simulink model "BigFour6sStEnCtrl"  (R2018b)
settings: Solver=FixedStepDiscrete  StartTime=0.0  StopTime=10.0  RelTol=1e-3
undefined symbols (not defined in the file or in its folder): data, KeSMSw4SSecRwLtStLgrstOtwdInwdClosePos1_Val, KeSMSw4SSecRwLtStLgrstUpwdDnwdClosePos1_Val, KeSMSw4SSecRwLtStLgrstUpwdDnwdClosePos2_Val, SecRwLtStBkReclnEn_Clear, SecRwLtStBkReclnEn_Set, SecRwLtStFwdBkwdEn_Clear, SecRwLtStFwdBkwdEn_Set, SecRwLtStLgrstInwdOtwdEn_Clear, SecRwLtStLgrstInwdOtwdEn_Set, SecRwLtStLgrstUpwdDnwdEn_Clear, SecRwLtStLgrstUpwdDnwdEn_Set, SecRwRtStBkReclnEn_Clear, SecRwRtStBkReclnEn_Set, SecRwRtStFwdBkwdEn_Clear, SecRwRtStFwdBkwdEn_Set, SecRwRtStLgrstInwdOtwdEn_Clear, SecRwRtStLgrstInwdOtwdEn_Set, SecRwRtStLgrstUpwdDnwdEn_Clear, SecRwRtStLgrstUpwdDnwdEn_Set, ThdRwLtStBkReclnEn_Clear, ThdRwLtStBkReclnEn_Set, ThdRwLtStFwdBkwdEn_Clear, ThdRwLtStFwdBkwdEn_Set, ThdRwRtStBkReclnEn_Clear, ThdRwRtStBkReclnEn_Set, ThdRwRtStFwdBkwdEn_Clear, ThdRwRtStFwdBkwdEn_Set, ZeroLEn_Clear, ZeroLEn_Set, ZeroREn_Clear, ZeroREn_Set
libraries: simulink x1
settings Model: Creator=sn2xws  LastModifiedBy=sn55gm
settings Model: ModifiedHistory=|
  | 2024.9.9 V3.0.0 新增Md56
  | 2024.9.26 V3.0.1 Md56流程从Md1复制
settings DataIOCC: SaveFormat=StructureWithTime
settings OptimizationCC: DefaultParameterBehavior=Inlined  EnhancedBackFolding=on  PassReuseOutputArgsAs=Individual arguments  ZeroExternalMemoryAtStartup=off  ZeroInternalMemoryAtStartup=off  OptimizeBlockOrder=speed  DifferentSizesBufferReuse=on  OptimizationCustomize=off
settings DebuggingCC: ParameterTunabilityLossMsg=error
settings SFSimCC: MATLABDynamicMemAlloc=off
settings RTWCC: SystemTargetFile=autosar.tlc  GenCodeOnly=on  TemplateMakefile=ert_default_tmf  Description=AUTOSAR  GenerateReport=on  IncludeHyperlinkInReport=on  LaunchReport=on  GenerateTraceInfo=on  GenerateTraceReport=on  GenerateTraceReportSl=on  GenerateTraceReportSf=on  GenerateTraceReportEml=on
settings CodeAppCC: ForceParamTrailComments=on  IgnoreCustomStorageClasses=off  OperatorAnnotations=on  SimulinkDataObjDesc=on  SFDataObjDesc=on  InsertBlockDesc=on
settings STFCustomTargetCC: TargetLangStandard=C99 (ISO)  MultiwordLength=256  ParMdlRefBuildCompliant=on  CompOptLevelCompliant=on  IncludeMdlTerminateFcn=off  CombineOutputUpdateFcns=on  SuppressErrorStatus=on  ERTCustomFileBanners=on  SupportNonFinite=off  SupportComplex=off  SupportContinuousTime=off  SupportNonInlinedSFcns=off  RemoveResetFunc=on  MATLABClassNameForMDSCustomization=Simulink.SoftwareTarget.ERTCustomization  AutosarCompliant=on  UseToolchainInfoCompliant=on  LookupTableObjectStructAxisOrder=2,1,3,4,...  LUTObjectStructOrderEvenSpacing=Size,Table,Breakpoints  SystemTargetFile=autosar.tlc
settings ERTTargetCC: TargetLangStandard=C99 (ISO)  ConcurrentExecutionCompliant=off  IncludeMdlTerminateFcn=off  SuppressErrorStatus=on  SupportNonFinite=off  SupportComplex=off  ModelStepFunctionPrototypeControlCompliant=off  CPPClassGenCompliant=off  AutosarCompliant=on  LookupTableObjectStructAxisOrder=2,1,3,4,...  LUTObjectStructOrderEvenSpacing=Size,Table,Breakpoints  InlinedParameterPlacement=NonHierarchical  ERTCustomFileTemplate=example_file_process.tlc  ERTFilePackagingFormat=Compact

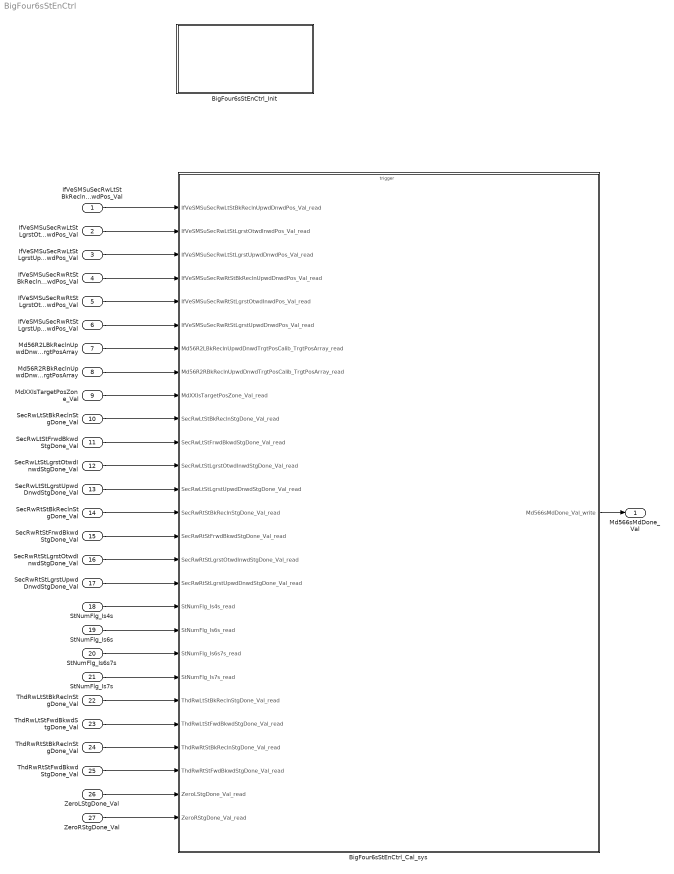
== system BigFour6sStEnCtrl ==
  IfVeSMSuSecRwLtStBkReclnUpwdDnwdPos_Val : Inport  OutDataTypeStr=uint16  PortDimensions=1
  IfVeSMSuSecRwLtStLgrstOtwdInwdPos_Val : Inport  Port=2  OutDataTypeStr=uint16  PortDimensions=1
  IfVeSMSuSecRwLtStLgrstUpwdDnwdPos_Val : Inport  Port=3  OutDataTypeStr=uint16  PortDimensions=1
  IfVeSMSuSecRwRtStBkReclnUpwdDnwdPos_Val : Inport  Port=4  OutDataTypeStr=uint16  PortDimensions=1
  IfVeSMSuSecRwRtStLgrstOtwdInwdPos_Val : Inport  Port=5  OutDataTypeStr=uint16  PortDimensions=1
  IfVeSMSuSecRwRtStLgrstUpwdDnwdPos_Val : Inport  Port=6  OutDataTypeStr=uint16  PortDimensions=1
  Md56R2LBkReclnUpwdDnwdTrgtPosCalib_TrgtPosArray : Inport  Description=|  Port=7  OutDataTypeStr=uint16  PortDimensions=3
      | 0:Pos
      | 1:Max
      | 2:Min
  Md56R2RBkReclnUpwdDnwdTrgtPosCalib_TrgtPosArray : Inport  Description=|  Port=8  OutDataTypeStr=uint16  PortDimensions=3
      | 0:Pos
      | 1:Max
      | 2:Min
  MdXXIsTargetPosZone_Val : Inport  Port=9  OutDataTypeStr=uint32  PortDimensions=1
  SecRwLtStBkReclnStgDone_Val : Inport  Port=10  OutDataTypeStr=boolean  PortDimensions=1
  SecRwLtStFrwdBkwdStgDone_Val : Inport  Port=11  OutDataTypeStr=boolean  PortDimensions=1
  SecRwLtStLgrstOtwdInwdStgDone_Val : Inport  Port=12  OutDataTypeStr=boolean  PortDimensions=1
  SecRwLtStLgrstUpwdDnwdStgDone_Val : Inport  Port=13  OutDataTypeStr=boolean  PortDimensions=1
  SecRwRtStBkReclnStgDone_Val : Inport  Port=14  OutDataTypeStr=boolean  PortDimensions=1
  SecRwRtStFrwdBkwdStgDone_Val : Inport  Port=15  OutDataTypeStr=boolean  PortDimensions=1
  SecRwRtStLgrstOtwdInwdStgDone_Val : Inport  Port=16  OutDataTypeStr=boolean  PortDimensions=1
  SecRwRtStLgrstUpwdDnwdStgDone_Val : Inport  Port=17  OutDataTypeStr=boolean  PortDimensions=1
  StNumFlg_Is4s : Inport  Port=18  OutDataTypeStr=boolean  PortDimensions=1
  StNumFlg_Is6s : Inport  Port=19  OutDataTypeStr=boolean  PortDimensions=1
  StNumFlg_Is6s7s : Inport  Port=20  OutDataTypeStr=boolean  PortDimensions=1
  StNumFlg_Is7s : Inport  Port=21  OutDataTypeStr=boolean  PortDimensions=1
  ThdRwLtStBkReclnStgDone_Val : Inport  Port=22  OutDataTypeStr=boolean  PortDimensions=1
  ThdRwLtStFwdBkwdStgDone_Val : Inport  Port=23  OutDataTypeStr=boolean  PortDimensions=1
  ThdRwRtStBkReclnStgDone_Val : Inport  Port=24  OutDataTypeStr=boolean  PortDimensions=1
  ThdRwRtStFwdBkwdStgDone_Val : Inport  Port=25  OutDataTypeStr=boolean  PortDimensions=1
  ZeroLStgDone_Val : Inport  Port=26  OutDataTypeStr=boolean  PortDimensions=1
  ZeroRStgDone_Val : Inport  Port=27  OutDataTypeStr=boolean  PortDimensions=1
  BigFour6sStEnCtrl_Cal_sys : Subsystem
  BigFour6sStEnCtrl_Init : Subsystem
  Md566sMdDone_Val : Outport  OutDataTypeStr=uint8  PortDimensions=1
  wires:
  IfVeSMSuSecRwLtStBkReclnUpwdDnwdPos_Val/1 -> BigFour6sStEnCtrl_Cal_sys/1(IfVeSMSuSecRwLtStBkReclnUpwdDnwdPos_Val_read)
  IfVeSMSuSecRwLtStLgrstOtwdInwdPos_Val/1 -> BigFour6sStEnCtrl_Cal_sys/2(IfVeSMSuSecRwLtStLgrstOtwdInwdPos_Val_read)
  IfVeSMSuSecRwLtStLgrstUpwdDnwdPos_Val/1 -> BigFour6sStEnCtrl_Cal_sys/3(IfVeSMSuSecRwLtStLgrstUpwdDnwdPos_Val_read)
  IfVeSMSuSecRwRtStBkReclnUpwdDnwdPos_Val/1 -> BigFour6sStEnCtrl_Cal_sys/4(IfVeSMSuSecRwRtStBkReclnUpwdDnwdPos_Val_read)
  IfVeSMSuSecRwRtStLgrstOtwdInwdPos_Val/1 -> BigFour6sStEnCtrl_Cal_sys/5(IfVeSMSuSecRwRtStLgrstOtwdInwdPos_Val_read)
  IfVeSMSuSecRwRtStLgrstUpwdDnwdPos_Val/1 -> BigFour6sStEnCtrl_Cal_sys/6(IfVeSMSuSecRwRtStLgrstUpwdDnwdPos_Val_read)
  Md56R2LBkReclnUpwdDnwdTrgtPosCalib_TrgtPosArray/1 -> BigFour6sStEnCtrl_Cal_sys/7(Md56R2LBkReclnUpwdDnwdTrgtPosCalib_TrgtPosArray_read)
  Md56R2RBkReclnUpwdDnwdTrgtPosCalib_TrgtPosArray/1 -> BigFour6sStEnCtrl_Cal_sys/8(Md56R2RBkReclnUpwdDnwdTrgtPosCalib_TrgtPosArray_read)
  MdXXIsTargetPosZone_Val/1 -> BigFour6sStEnCtrl_Cal_sys/9(MdXXIsTargetPosZone_Val_read)
  SecRwLtStBkReclnStgDone_Val/1 -> BigFour6sStEnCtrl_Cal_sys/10(SecRwLtStBkReclnStgDone_Val_read)
  SecRwLtStFrwdBkwdStgDone_Val/1 -> BigFour6sStEnCtrl_Cal_sys/11(SecRwLtStFrwdBkwdStgDone_Val_read)
  SecRwLtStLgrstOtwdInwdStgDone_Val/1 -> BigFour6sStEnCtrl_Cal_sys/12(SecRwLtStLgrstOtwdInwdStgDone_Val_read)
  SecRwLtStLgrstUpwdDnwdStgDone_Val/1 -> BigFour6sStEnCtrl_Cal_sys/13(SecRwLtStLgrstUpwdDnwdStgDone_Val_read)
  SecRwRtStBkReclnStgDone_Val/1 -> BigFour6sStEnCtrl_Cal_sys/14(SecRwRtStBkReclnStgDone_Val_read)
  SecRwRtStFrwdBkwdStgDone_Val/1 -> BigFour6sStEnCtrl_Cal_sys/15(SecRwRtStFrwdBkwdStgDone_Val_read)
  SecRwRtStLgrstOtwdInwdStgDone_Val/1 -> BigFour6sStEnCtrl_Cal_sys/16(SecRwRtStLgrstOtwdInwdStgDone_Val_read)
  SecRwRtStLgrstUpwdDnwdStgDone_Val/1 -> BigFour6sStEnCtrl_Cal_sys/17(SecRwRtStLgrstUpwdDnwdStgDone_Val_read)
  StNumFlg_Is4s/1 -> BigFour6sStEnCtrl_Cal_sys/18(StNumFlg_Is4s_read)
  StNumFlg_Is6s/1 -> BigFour6sStEnCtrl_Cal_sys/19(StNumFlg_Is6s_read)
  StNumFlg_Is6s7s/1 -> BigFour6sStEnCtrl_Cal_sys/20(StNumFlg_Is6s7s_read)
  StNumFlg_Is7s/1 -> BigFour6sStEnCtrl_Cal_sys/21(StNumFlg_Is7s_read)
  ThdRwLtStBkReclnStgDone_Val/1 -> BigFour6sStEnCtrl_Cal_sys/22(ThdRwLtStBkReclnStgDone_Val_read)
  ThdRwLtStFwdBkwdStgDone_Val/1 -> BigFour6sStEnCtrl_Cal_sys/23(ThdRwLtStFwdBkwdStgDone_Val_read)
  ThdRwRtStBkReclnStgDone_Val/1 -> BigFour6sStEnCtrl_Cal_sys/24(ThdRwRtStBkReclnStgDone_Val_read)
  ThdRwRtStFwdBkwdStgDone_Val/1 -> BigFour6sStEnCtrl_Cal_sys/25(ThdRwRtStFwdBkwdStgDone_Val_read)
  ZeroLStgDone_Val/1 -> BigFour6sStEnCtrl_Cal_sys/26(ZeroLStgDone_Val_read)
  ZeroRStgDone_Val/1 -> BigFour6sStEnCtrl_Cal_sys/27(ZeroRStgDone_Val_read)
  BigFour6sStEnCtrl_Cal_sys/1(Md566sMdDone_Val_write) -> Md566sMdDone_Val/1

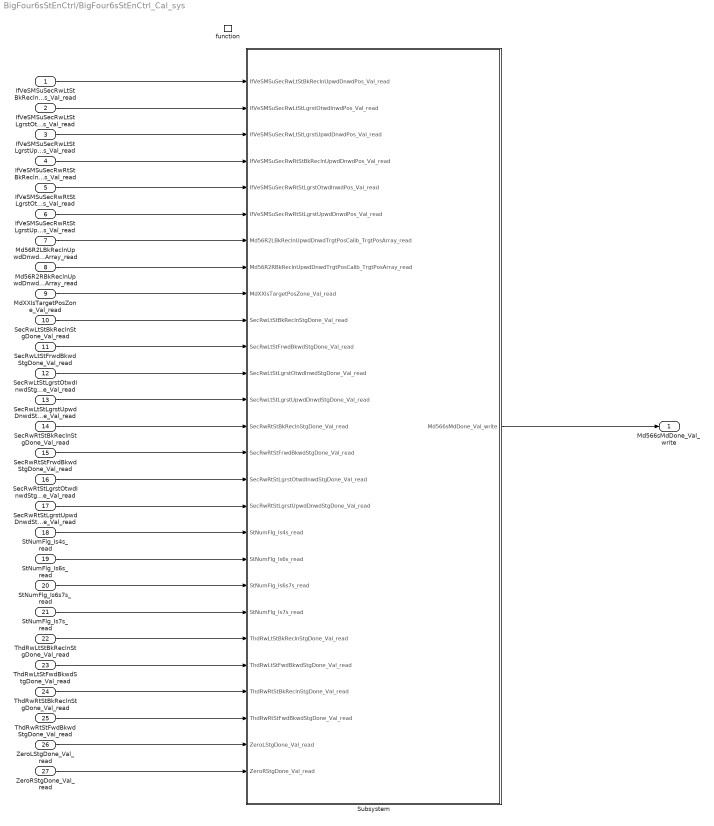
== system BigFour6sStEnCtrl/BigFour6sStEnCtrl_Cal_sys ==
  IfVeSMSuSecRwLtStBkReclnUpwdDnwdPos_Val_read : Inport
  IfVeSMSuSecRwLtStLgrstOtwdInwdPos_Val_read : Inport  Port=2
  IfVeSMSuSecRwLtStLgrstUpwdDnwdPos_Val_read : Inport  Port=3
  IfVeSMSuSecRwRtStBkReclnUpwdDnwdPos_Val_read : Inport  Port=4
  IfVeSMSuSecRwRtStLgrstOtwdInwdPos_Val_read : Inport  Port=5
  IfVeSMSuSecRwRtStLgrstUpwdDnwdPos_Val_read : Inport  Port=6
  Md56R2LBkReclnUpwdDnwdTrgtPosCalib_TrgtPosArray_read : Inport  Port=7
  Md56R2RBkReclnUpwdDnwdTrgtPosCalib_TrgtPosArray_read : Inport  Port=8
  MdXXIsTargetPosZone_Val_read : Inport  Port=9
  SecRwLtStBkReclnStgDone_Val_read : Inport  Port=10
  SecRwLtStFrwdBkwdStgDone_Val_read : Inport  Port=11
  SecRwLtStLgrstOtwdInwdStgDone_Val_read : Inport  Port=12
  SecRwLtStLgrstUpwdDnwdStgDone_Val_read : Inport  Port=13
  SecRwRtStBkReclnStgDone_Val_read : Inport  Port=14
  SecRwRtStFrwdBkwdStgDone_Val_read : Inport  Port=15
  SecRwRtStLgrstOtwdInwdStgDone_Val_read : Inport  Port=16
  SecRwRtStLgrstUpwdDnwdStgDone_Val_read : Inport  Port=17
  StNumFlg_Is4s_read : Inport  Port=18
  StNumFlg_Is6s_read : Inport  Port=19
  StNumFlg_Is6s7s_read : Inport  Port=20
  StNumFlg_Is7s_read : Inport  Port=21
  ThdRwLtStBkReclnStgDone_Val_read : Inport  Port=22
  ThdRwLtStFwdBkwdStgDone_Val_read : Inport  Port=23
  ThdRwRtStBkReclnStgDone_Val_read : Inport  Port=24
  ThdRwRtStFwdBkwdStgDone_Val_read : Inport  Port=25
  ZeroLStgDone_Val_read : Inport  Port=26
  ZeroRStgDone_Val_read : Inport  Port=27
  function : TriggerPort  TriggerType=function-call  IsSimulinkFunction=on  FunctionName=BigFour6sStEnCtrl_Cal  VariantControl=(inherit)
  Subsystem : Subsystem
  Md566sMdDone_Val_write : Outport
      settings: EnsureOutportIsVirtual=on
  wires:
  IfVeSMSuSecRwLtStBkReclnUpwdDnwdPos_Val_read/1 -> Subsystem/1(IfVeSMSuSecRwLtStBkReclnUpwdDnwdPos_Val_read)
  IfVeSMSuSecRwLtStLgrstOtwdInwdPos_Val_read/1 -> Subsystem/2(IfVeSMSuSecRwLtStLgrstOtwdInwdPos_Val_read)
  IfVeSMSuSecRwLtStLgrstUpwdDnwdPos_Val_read/1 -> Subsystem/3(IfVeSMSuSecRwLtStLgrstUpwdDnwdPos_Val_read)
  IfVeSMSuSecRwRtStBkReclnUpwdDnwdPos_Val_read/1 -> Subsystem/4(IfVeSMSuSecRwRtStBkReclnUpwdDnwdPos_Val_read)
  IfVeSMSuSecRwRtStLgrstOtwdInwdPos_Val_read/1 -> Subsystem/5(IfVeSMSuSecRwRtStLgrstOtwdInwdPos_Val_read)
  IfVeSMSuSecRwRtStLgrstUpwdDnwdPos_Val_read/1 -> Subsystem/6(IfVeSMSuSecRwRtStLgrstUpwdDnwdPos_Val_read)
  Md56R2LBkReclnUpwdDnwdTrgtPosCalib_TrgtPosArray_read/1 -> Subsystem/7(Md56R2LBkReclnUpwdDnwdTrgtPosCalib_TrgtPosArray_read)
  Md56R2RBkReclnUpwdDnwdTrgtPosCalib_TrgtPosArray_read/1 -> Subsystem/8(Md56R2RBkReclnUpwdDnwdTrgtPosCalib_TrgtPosArray_read)
  MdXXIsTargetPosZone_Val_read/1 -> Subsystem/9(MdXXIsTargetPosZone_Val_read)
  SecRwLtStBkReclnStgDone_Val_read/1 -> Subsystem/10(SecRwLtStBkReclnStgDone_Val_read)
  SecRwLtStFrwdBkwdStgDone_Val_read/1 -> Subsystem/11(SecRwLtStFrwdBkwdStgDone_Val_read)
  SecRwLtStLgrstOtwdInwdStgDone_Val_read/1 -> Subsystem/12(SecRwLtStLgrstOtwdInwdStgDone_Val_read)
  SecRwLtStLgrstUpwdDnwdStgDone_Val_read/1 -> Subsystem/13(SecRwLtStLgrstUpwdDnwdStgDone_Val_read)
  SecRwRtStBkReclnStgDone_Val_read/1 -> Subsystem/14(SecRwRtStBkReclnStgDone_Val_read)
  SecRwRtStFrwdBkwdStgDone_Val_read/1 -> Subsystem/15(SecRwRtStFrwdBkwdStgDone_Val_read)
  SecRwRtStLgrstOtwdInwdStgDone_Val_read/1 -> Subsystem/16(SecRwRtStLgrstOtwdInwdStgDone_Val_read)
  SecRwRtStLgrstUpwdDnwdStgDone_Val_read/1 -> Subsystem/17(SecRwRtStLgrstUpwdDnwdStgDone_Val_read)
  StNumFlg_Is4s_read/1 -> Subsystem/18(StNumFlg_Is4s_read)
  StNumFlg_Is6s_read/1 -> Subsystem/19(StNumFlg_Is6s_read)
  StNumFlg_Is6s7s_read/1 -> Subsystem/20(StNumFlg_Is6s7s_read)
  StNumFlg_Is7s_read/1 -> Subsystem/21(StNumFlg_Is7s_read)
  ThdRwLtStBkReclnStgDone_Val_read/1 -> Subsystem/22(ThdRwLtStBkReclnStgDone_Val_read)
  ThdRwLtStFwdBkwdStgDone_Val_read/1 -> Subsystem/23(ThdRwLtStFwdBkwdStgDone_Val_read)
  ThdRwRtStBkReclnStgDone_Val_read/1 -> Subsystem/24(ThdRwRtStBkReclnStgDone_Val_read)
  ThdRwRtStFwdBkwdStgDone_Val_read/1 -> Subsystem/25(ThdRwRtStFwdBkwdStgDone_Val_read)
  ZeroLStgDone_Val_read/1 -> Subsystem/26(ZeroLStgDone_Val_read)
  ZeroRStgDone_Val_read/1 -> Subsystem/27(ZeroRStgDone_Val_read)
  Subsystem/1(Md566sMdDone_Val_write) -> Md566sMdDone_Val_write/1

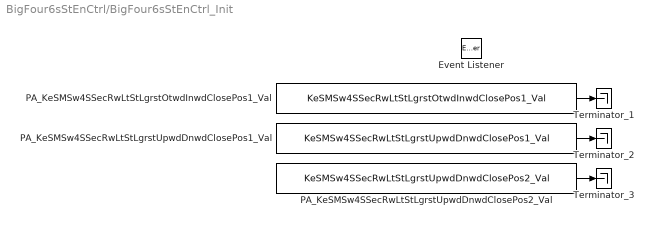
== system BigFour6sStEnCtrl/BigFour6sStEnCtrl_Init ==
  Event Listener : EventListener  EventName=reset
  PA_KeSMSw4SSecRwLtStLgrstOtwdInwdClosePos1_Val : Constant  Value=KeSMSw4SSecRwLtStLgrstOtwdInwdClosePos1_Val
  PA_KeSMSw4SSecRwLtStLgrstUpwdDnwdClosePos1_Val : Constant  Value=KeSMSw4SSecRwLtStLgrstUpwdDnwdClosePos1_Val
  PA_KeSMSw4SSecRwLtStLgrstUpwdDnwdClosePos2_Val : Constant  Value=KeSMSw4SSecRwLtStLgrstUpwdDnwdClosePos2_Val
  Terminator_1 : Terminator
  Terminator_2 : Terminator
  Terminator_3 : Terminator
  wires:
  PA_KeSMSw4SSecRwLtStLgrstOtwdInwdClosePos1_Val/1 -> Terminator_1/1
  PA_KeSMSw4SSecRwLtStLgrstUpwdDnwdClosePos1_Val/1 -> Terminator_2/1
  PA_KeSMSw4SSecRwLtStLgrstUpwdDnwdClosePos2_Val/1 -> Terminator_3/1

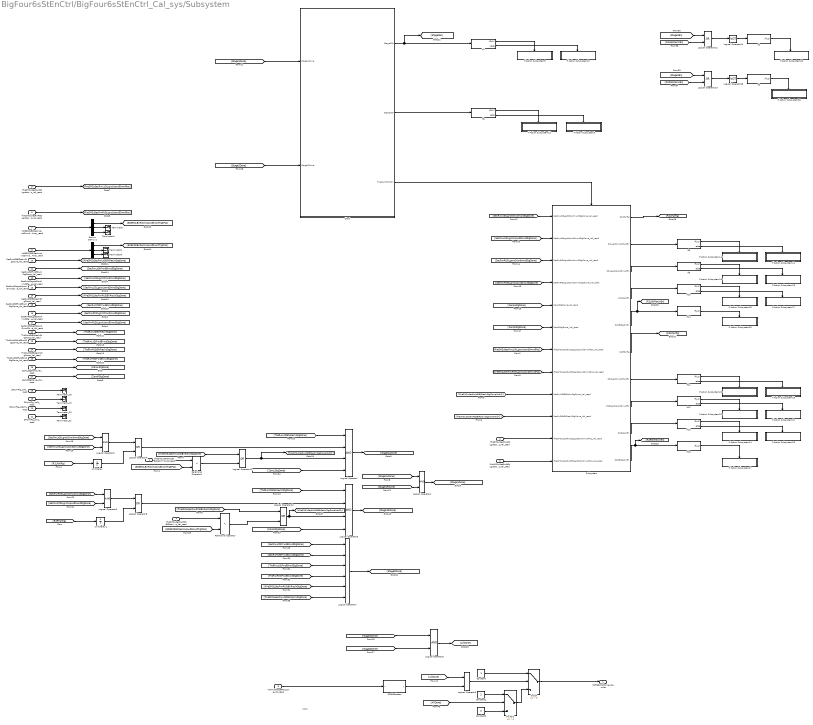
== system BigFour6sStEnCtrl/BigFour6sStEnCtrl_Cal_sys/Subsystem ==
  note: Md56
  IfVeSMSuSecRwLtStBkReclnUpwdDnwdPos_Val_read : Inport
  IfVeSMSuSecRwLtStLgrstOtwdInwdPos_Val_read : Inport  Port=2
  IfVeSMSuSecRwLtStLgrstUpwdDnwdPos_Val_read : Inport  Port=3
  IfVeSMSuSecRwRtStBkReclnUpwdDnwdPos_Val_read : Inport  Port=4
  IfVeSMSuSecRwRtStLgrstOtwdInwdPos_Val_read : Inport  Port=5
  IfVeSMSuSecRwRtStLgrstUpwdDnwdPos_Val_read : Inport  Port=6
  Md56R2LBkReclnUpwdDnwdTrgtPosCalib_TrgtPosArray_read : Inport  Port=7
  Md56R2RBkReclnUpwdDnwdTrgtPosCalib_TrgtPosArray_read : Inport  Port=8
  MdXXIsTargetPosZone_Val_read : Inport  Port=9
  SecRwLtStBkReclnStgDone_Val_read : Inport  Port=10
  SecRwLtStFrwdBkwdStgDone_Val_read : Inport  Port=11
  SecRwLtStLgrstOtwdInwdStgDone_Val_read : Inport  Port=12
  SecRwLtStLgrstUpwdDnwdStgDone_Val_read : Inport  Port=13
  SecRwRtStBkReclnStgDone_Val_read : Inport  Port=14
  SecRwRtStFrwdBkwdStgDone_Val_read : Inport  Port=15
  SecRwRtStLgrstOtwdInwdStgDone_Val_read : Inport  Port=16
  SecRwRtStLgrstUpwdDnwdStgDone_Val_read : Inport  Port=17
  StNumFlg_Is4s_read : Inport  Port=18
  StNumFlg_Is6s_read : Inport  Port=19
  StNumFlg_Is6s7s_read : Inport  Port=20
  StNumFlg_Is7s_read : Inport  Port=21
  ThdRwLtStBkReclnStgDone_Val_read : Inport  Port=22
  ThdRwLtStFwdBkwdStgDone_Val_read : Inport  Port=23
  ThdRwRtStBkReclnStgDone_Val_read : Inport  Port=24
  ThdRwRtStFwdBkwdStgDone_Val_read : Inport  Port=25
  ZeroLStgDone_Val_read : Inport  Port=26
  ZeroRStgDone_Val_read : Inport  Port=27
  32BitSelector : Subsystem  mask(32 Bit Selector){BitNum=24}
      mask prompts: BitNum "Select Bit Number"
      mask help: Allows selection of a particular bit (0-31) out of a packed word up to 32 bits long. Output will be true if the bit number selected via the mask parameter is equal to one.
      mask TypeOptions BitNum: 0 | 1 | 2 | 3 | 4 | 5 | 6 | 7 | 8 | 9 | 10 | 11 | 12 | 13 | 14 | 15 | 16 | 17 | 18 | 19 | 20 | 21 | 22 | 23 | 24 | 25 | 26 | 27 | 28 | 29 | 30 | 31
      mask Display:
      | text(0.5, 0.8,'BIT','horizontalAlignment','center')
      | text(0.5, 0.5,'SELECTOR','horizontalAlignment','center')
      | text(0.5, 0.2,['-- Bit ',char(get_param(gcb,'BitNum')),' --'],'horizontalAlignment','center')
  Chart : Stateflow chart  TreatAsAtomicUnit=on
  Constant : Constant  OutDataTypeStr=uint8
  Constant1 : Constant  Value=2  OutDataTypeStr=uint8
  Constant2 : Constant  Value=0  OutDataTypeStr=uint8
  Demux : Demux  Outputs=3
  Demux1 : Demux  Outputs=3
  If Action Subsystem10 : Subsystem  TreatAsAtomicUnit=on
  If Action Subsystem11 : Subsystem  TreatAsAtomicUnit=on
  If Action Subsystem12 : Subsystem  TreatAsAtomicUnit=on
  If Action Subsystem14 : Subsystem  TreatAsAtomicUnit=on
  If Action Subsystem15 : Subsystem  TreatAsAtomicUnit=on
  If Action Subsystem16 : Subsystem  TreatAsAtomicUnit=on
  If Action Subsystem17 : Subsystem  TreatAsAtomicUnit=on
  If Action Subsystem18 : Subsystem  TreatAsAtomicUnit=on
  If Action Subsystem19 : Subsystem  TreatAsAtomicUnit=on
  If Action Subsystem20 : Subsystem  TreatAsAtomicUnit=on
  If Action Subsystem21 : Subsystem  TreatAsAtomicUnit=on
  If Action Subsystem22 : Subsystem  TreatAsAtomicUnit=on
  If Action Subsystem23 : Subsystem  TreatAsAtomicUnit=on
  If Action Subsystem24 : Subsystem  TreatAsAtomicUnit=on
  If Action Subsystem25 : Subsystem  TreatAsAtomicUnit=on
  If Action Subsystem26 : Subsystem  TreatAsAtomicUnit=on
  If Action Subsystem27 : Subsystem  TreatAsAtomicUnit=on
  If Action Subsystem28 : Subsystem  TreatAsAtomicUnit=on
  If Action Subsystem3 : Subsystem  TreatAsAtomicUnit=on
  If Action Subsystem9 : Subsystem  TreatAsAtomicUnit=on
  If{1..2,14..15} (4 alike) : If  IfExpression=u1  ShowElse=off
  If{6..13} (8 alike) : If  IfExpression=u1
  Logical Operator : Logic  Inputs=4  AllPortsSameDT=off  OutDataTypeStr=boolean
  Logical Operator{1..2,5..6,9} (5 alike) : Logic  AllPortsSameDT=off  OutDataTypeStr=boolean
  Logical Operator{4,8,10..13} (6 alike) : Logic  Operator=OR  AllPortsSameDT=off  OutDataTypeStr=boolean
  Logical Operator14 : Logic  Operator=NOT  AllPortsSameDT=off  OutDataTypeStr=boolean
  Logical Operator15 : Logic  Operator=NOT  AllPortsSameDT=off  OutDataTypeStr=boolean
  Logical Operator3 : Logic  Inputs=4  AllPortsSameDT=off  OutDataTypeStr=boolean
  Logical Operator7 : Logic  Inputs=6  AllPortsSameDT=off  OutDataTypeStr=boolean
  Relational Operator : RelationalOperator  Operator=<  OutDataTypeStr=boolean  RndMeth=Simplest
  Relational Operator1 : RelationalOperator  Operator=<  OutDataTypeStr=boolean  RndMeth=Simplest
  Subsystem : Subsystem
  Switch : Switch  Criteria=u2 > Threshold
  Switch1 : Switch  Criteria=u2 > Threshold
  Terminator{,1..3} (4 alike) : Terminator
  Terminator_{18..21} (4 alike) : Terminator
  Unit Delay : UnitDelay  SampleTime=-1
  Unit Delay1 : UnitDelay  SampleTime=-1
  Md566sMdDone_Val_write : Outport
      settings: EnsureOutportIsVirtual=on
  wires:
  StNumFlg_Is7s_read/1 -> Terminator_21/1
  StNumFlg_Is6s7s_read/1 -> Terminator_20/1
  StNumFlg_Is4s_read/1 -> Terminator_18/1
  StNumFlg_Is6s_read/1 -> Terminator_19/1
  Logical Operator9/1 -> Switch/2
  Switch1/1 -> Switch/3
  [AllDone] -> Logical Operator9/1
  Constant1/1 -> Switch1/1
  [AllDone] -> Switch1/2
  32BitSelector/1(y) -> Logical Operator9/2
  Constant2/1 -> Switch1/3
  Switch/1 -> Md566sMdDone_Val_write/1
  MdXXIsTargetPosZone_Val_read/1 -> 32BitSelector/1(x)
  Constant/1 -> Switch/1
  [Stage2Done] -> Logical Operator5/2
  Logical Operator5/1 -> [AllDone]
  [Stage1Done] -> Logical Operator5/1
  [SecRwRtStLgrstUpwdDnwdStgDone] -> Subsystem/4(SecRwRtStLgrstUpwdDnwdStgDone_Val_read)
  If9/2 -> If Action Subsystem15/Action
  Subsystem/6(R2RFailflg) -> [R2RFailflg]
  [IfVeSMSuSecRwRtStBkReclnStgDoneModify] -> Subsystem/10(SecRwRtStBkReclnStgDone_Val_read)
  If12/1 -> If Action Subsystem22/Action
  Subsystem/5(R2LBkReclnEn) -> [R2LBkReclnEn], If14/1
  If13/1 -> If Action Subsystem24/Action
  [IfVeSMSuSecRwRtStLgrstUpwdDnwdPos] -> Subsystem/8(IfVeSMSuSecRwRtStLgrstUpwdDnwdPos_Val_read)
  If11/1 -> If Action Subsystem20/Action
  [SecRwLtStLgrstOtwdInwdStgDone] -> Subsystem/1(SecRwLtStLgrstOtwdInwdStgDone_Val_read)
  [SecRwRtStLgrstOtwdInwdStgDone] -> Subsystem/3(SecRwRtStLgrstOtwdInwdStgDone_Val_read)
  If14/1 -> If Action Subsystem25/Action
  If9/1 -> If Action Subsystem16/Action
  Subsystem/3(R2LLgrstUpwdDnwdEn) -> If9/1
  Chart/3(TrigComfortMd()) -> Subsystem/Trigger
  If8/2 -> If Action Subsystem11/Action
  Subsystem/9(R2RZeroEn) -> If13/1
  If13/2 -> If Action Subsystem23/Action
  If12/2 -> If Action Subsystem21/Action
  Subsystem/1(R2LFailflg) -> [R2LFailflg]
  If11/2 -> If Action Subsystem19/Action
  Subsystem/2(R2LLgrstInwdOtwdEn) -> If8/1
  Subsystem/4(R2LZeroEn) -> If10/1
  If8/1 -> If Action Subsystem14/Action
  Subsystem/8(R2RLgrstUpwdDnwdEn) -> If12/1
  [IfVeSMSuSecRwLtStLgrstUpwdDnwdPos] -> Subsystem/7(IfVeSMSuSecRwLtStLgrstUpwdDnwdPos_Val_read)
  Subsystem/7(R2RLgrstInwdOtwdEn) -> If11/1
  [ZeroRStgDone] -> Subsystem/6(ZeroRStgDone_Val_read)
  [ZeroLStgDone] -> Subsystem/5(ZeroLStgDone_Val_read)
  Subsystem/10(R2RBkReclnEn) -> [R2RBkReclnEn], If15/1
  If15/1 -> If Action Subsystem27/Action
  If10/1 -> If Action Subsystem18/Action
  If10/2 -> If Action Subsystem17/Action
  [SecRwLtStLgrstUpwdDnwdStgDone] -> Subsystem/2(SecRwLtStLgrstUpwdDnwdStgDone_Val_read)
  [IfVeSMSuSecRwLtStBkReclnStgDoneModify] -> Subsystem/9(SecRwLtStBkReclnStgDone_Val_read)
  If6/2 -> If Action Subsystem3/Action
  If7/1 -> If Action Subsystem9/Action
  Chart/1(Stage2En) -> [Stage2En], If7/1
  [Stage2En] -> Logical Operator13/1
  If1/1 -> If Action Subsystem26/Action
  Logical Operator14/1 -> If1/1
  Logical Operator13/1 -> Logical Operator15/1
  [Stage2En] -> Logical Operator12/1
  Logical Operator12/1 -> Logical Operator14/1
  If6/1 -> If Action Subsystem12/Action
  Chart/2(Stage1En) -> If6/1
  Logical Operator15/1 -> If2/1
  [R2LBkReclnEn] -> Logical Operator12/2
  If2/1 -> If Action Subsystem28/Action
  If7/2 -> If Action Subsystem10/Action
  [R2RBkReclnEn] -> Logical Operator13/2
  ThdRwLtStBkReclnStgDone_Val_read/1 -> [ThdRwLtStBkReclnStgDone]
  ThdRwRtStBkReclnStgDone_Val_read/1 -> [ThdRwRtStBkReclnStgDone]
  Md56R2LBkReclnUpwdDnwdTrgtPosCalib_TrgtPosArray_read/1 -> Demux/1
  Demux/1 -> [EZER2LBkReclnUpwdDnwdTrgtPos]
  Demux/3 -> Terminator1/1
  Demux1/2 -> Terminator2/1
  Demux1/3 -> Terminator3/1
  Demux1/1 -> [EZER2RBkReclnUpwdDnwdTrgtPos]
  ThdRwLtStFwdBkwdStgDone_Val_read/1 -> [ThdRwLtStFwdBkwdStgDone]
  Md56R2RBkReclnUpwdDnwdTrgtPosCalib_TrgtPosArray_read/1 -> Demux1/1
  Demux/2 -> Terminator/1
  IfVeSMSuSecRwLtStLgrstUpwdDnwdPos_Val_read/1 -> [IfVeSMSuSecRwLtStLgrstUpwdDnwdPos]
  IfVeSMSuSecRwRtStLgrstUpwdDnwdPos_Val_read/1 -> [IfVeSMSuSecRwRtStLgrstUpwdDnwdPos]
  SecRwLtStFrwdBkwdStgDone_Val_read/1 -> [SecRwLtStFrwdBkwdStgDone]
  SecRwLtStLgrstUpwdDnwdStgDone_Val_read/1 -> [SecRwLtStLgrstUpwdDnwdStgDone]
  SecRwRtStBkReclnStgDone_Val_read/1 -> [IfVeSMSuSecRwRtStBkReclnStgDone]
  SecRwRtStFrwdBkwdStgDone_Val_read/1 -> [SecRwRtStFrwdBkwdStgDone]
  SecRwRtStLgrstOtwdInwdStgDone_Val_read/1 -> [SecRwRtStLgrstOtwdInwdStgDone]
  SecRwRtStLgrstUpwdDnwdStgDone_Val_read/1 -> [SecRwRtStLgrstUpwdDnwdStgDone]
  ZeroLStgDone_Val_read/1 -> [ZeroLStgDone]
  ZeroRStgDone_Val_read/1 -> [ZeroRStgDone]
  ThdRwRtStFwdBkwdStgDone_Val_read/1 -> [ThdRwRtStFwdBkwdStgDone]
  SecRwLtStBkReclnStgDone_Val_read/1 -> [IfVeSMSuSecRwLtStBkReclnStgDone]
  SecRwLtStLgrstOtwdInwdStgDone_Val_read/1 -> [SecRwLtStLgrstOtwdInwdStgDone]
  IfVeSMSuSecRwLtStLgrstOtwdInwdPos_Val_read/1 -> Subsystem/11(IfVeSMSuSecRwLtStLgrstOtwdInwdPos_Val_read)
  IfVeSMSuSecRwRtStLgrstOtwdInwdPos_Val_read/1 -> Subsystem/12(IfVeSMSuSecRwRtStLgrstOtwdInwdPos_Val_read)
  [SecRwRtStLgrstUpwdDnwdStgDone] -> Logical Operator6/2
  [EZER2RBkReclnUpwdDnwdTrgtPos] -> Relational Operator/2
  Logical Operator6/1 -> Logical Operator8/1
  [R2LFailflg] -> Unit Delay/1
  Logical Operator11/1 -> [IfVeSMSuSecRwLtStBkReclnStgDoneModify], Logical Operator/3
  Logical Operator8/1 -> Logical Operator3/2
  [EZER2LBkReclnUpwdDnwdTrgtPos] -> Relational Operator1/2
  Logical Operator7/1 -> [Stage2Done]
  Logical Operator10/1 -> [IfVeSMSuSecRwRtStBkReclnStgDoneModify], Logical Operator3/3
  [IfVeSMSuSecRwLtStBkReclnStgDone] -> Logical Operator7/6
  Unit Delay1/1 -> Logical Operator8/2
  [SecRwRtStLgrstOtwdInwdStgDone] -> Logical Operator6/1
  [IfVeSMSuSecRwRtStBkReclnStgDone] -> Logical Operator7/5
  Logical Operator4/1 -> Logical Operator/2
  IfVeSMSuSecRwLtStBkReclnUpwdDnwdPos_Val_read/1 -> Relational Operator1/1
  [ThdRwLtStFwdBkwdStgDone] -> Logical Operator7/3
  Relational Operator/1 -> Logical Operator10/2
  [ThdRwRtStBkReclnStgDone] -> Logical Operator3/1
  IfVeSMSuSecRwRtStBkReclnUpwdDnwdPos_Val_read/1 -> Relational Operator/1
  Relational Operator1/1 -> Logical Operator11/2
  [Stage1LDone] -> Logical Operator1/1
  [IfVeSMSuSecRwRtStBkReclnStgDone] -> Logical Operator10/1
  [SecRwLtStLgrstUpwdDnwdStgDone] -> Logical Operator2/2
  [IfVeSMSuSecRwLtStBkReclnStgDone] -> Logical Operator11/1
  Unit Delay/1 -> Logical Operator4/2
  [ZeroRStgDone] -> Logical Operator3/4
  [R2RFailflg] -> Unit Delay1/1
  [Stage1RDone] -> Logical Operator1/2
  Logical Operator2/1 -> Logical Operator4/1
  [SecRwLtStLgrstOtwdInwdStgDone] -> Logical Operator2/1
  [ThdRwLtStBkReclnStgDone] -> Logical Operator/1
  Logical Operator/1 -> [Stage1LDone]
  [ThdRwRtStFwdBkwdStgDone] -> Logical Operator7/4
  [SecRwRtStFrwdBkwdStgDone] -> Logical Operator7/2
  [SecRwLtStFrwdBkwdStgDone] -> Logical Operator7/1
  Logical Operator3/1 -> [Stage1RDone]
  Logical Operator1/1 -> [Stage1Done]
  [ZeroLStgDone] -> Logical Operator/4
  [Stage2Done] -> Chart/2(Stage2Done)
  [Stage1Done] -> Chart/1(Stage1Done)

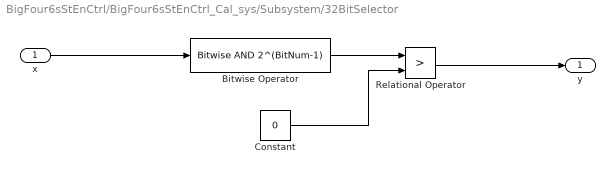
== system BigFour6sStEnCtrl/BigFour6sStEnCtrl_Cal_sys/Subsystem/32BitSelector ==
  x : Inport
  Bitwise Operator : simulink/Logic and Bit Operations/Bitwise Operator  logicop=AND  UseBitMask=on  BitMask=2^(BitNum-1)  BitMaskRealWorld=Stored Integer
  Constant : Constant  Value=0  OutDataTypeStr=uint32
  Relational Operator : RelationalOperator  Operator=>  OutDataTypeStr=boolean  RndMeth=Simplest
  y : Outport
  wires:
  Relational Operator/1 -> y/1
  Constant/1 -> Relational Operator/2
  x/1 -> Bitwise Operator/1
  Bitwise Operator/1 -> Relational Operator/1

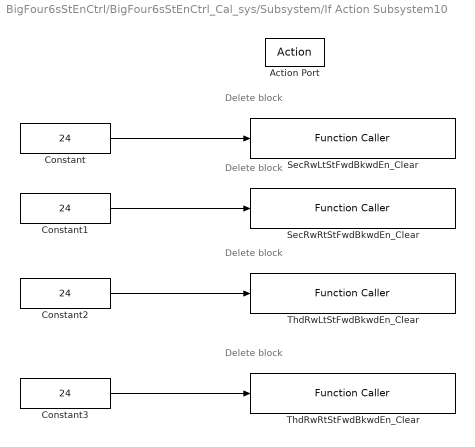
== system BigFour6sStEnCtrl/BigFour6sStEnCtrl_Cal_sys/Subsystem/If Action Subsystem10 ==
  note: Delete block
  note: Delete block
  note: Delete block
  note: Delete block
  Action Port : ActionPort  ActionType=else
  Constant{,1..3} (4 alike) : Constant  Value=24  OutDataTypeStr=uint8
  SecRwLtStFwdBkwdEn_Clear : FunctionCaller  FunctionPrototype=SecRwLtStFwdBkwdEn_Clear(data)  InputArgumentSpecifications=uint8(1)
  SecRwRtStFwdBkwdEn_Clear : FunctionCaller  FunctionPrototype=SecRwRtStFwdBkwdEn_Clear(data)  InputArgumentSpecifications=uint8(1)
  ThdRwLtStFwdBkwdEn_Clear : FunctionCaller  FunctionPrototype=ThdRwLtStFwdBkwdEn_Clear(data)  InputArgumentSpecifications=uint8(1)
  ThdRwRtStFwdBkwdEn_Clear : FunctionCaller  FunctionPrototype=ThdRwRtStFwdBkwdEn_Clear(data)  InputArgumentSpecifications=uint8(1)
  wires:
  Constant/1 -> SecRwLtStFwdBkwdEn_Clear/1
  Constant1/1 -> SecRwRtStFwdBkwdEn_Clear/1
  Constant2/1 -> ThdRwLtStFwdBkwdEn_Clear/1
  Constant3/1 -> ThdRwRtStFwdBkwdEn_Clear/1

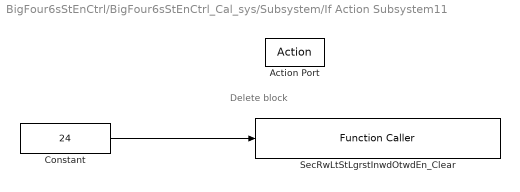
== system BigFour6sStEnCtrl/BigFour6sStEnCtrl_Cal_sys/Subsystem/If Action Subsystem11 ==
  note: Delete block
  Action Port : ActionPort  ActionType=else
  Constant : Constant  Value=24  OutDataTypeStr=uint8
  SecRwLtStLgrstInwdOtwdEn_Clear : FunctionCaller  FunctionPrototype=SecRwLtStLgrstInwdOtwdEn_Clear(data)  InputArgumentSpecifications=uint8(1)
  wires:
  Constant/1 -> SecRwLtStLgrstInwdOtwdEn_Clear/1

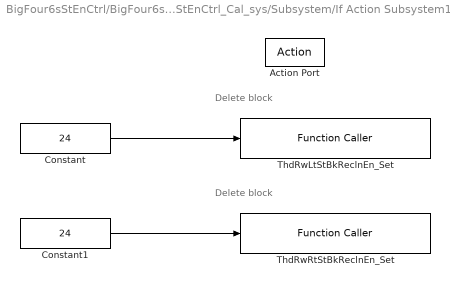
== system BigFour6sStEnCtrl/BigFour6sStEnCtrl_Cal_sys/Subsystem/If Action Subsystem12 ==
  note: Delete block
  note: Delete block
  Action Port : ActionPort  ActionType=then
  Constant : Constant  Value=24  OutDataTypeStr=uint8
  Constant1 : Constant  Value=24  OutDataTypeStr=uint8
  ThdRwLtStBkReclnEn_Set : FunctionCaller  FunctionPrototype=ThdRwLtStBkReclnEn_Set(data)  InputArgumentSpecifications=uint8(1)
  ThdRwRtStBkReclnEn_Set : FunctionCaller  FunctionPrototype=ThdRwRtStBkReclnEn_Set(data)  InputArgumentSpecifications=uint8(1)
  wires:
  Constant/1 -> ThdRwLtStBkReclnEn_Set/1
  Constant1/1 -> ThdRwRtStBkReclnEn_Set/1

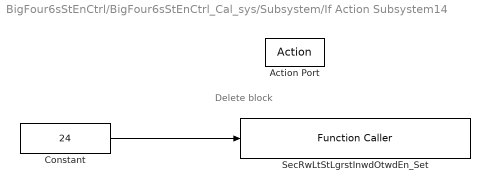
== system BigFour6sStEnCtrl/BigFour6sStEnCtrl_Cal_sys/Subsystem/If Action Subsystem14 ==
  note: Delete block
  Action Port : ActionPort  ActionType=then
  Constant : Constant  Value=24  OutDataTypeStr=uint8
  SecRwLtStLgrstInwdOtwdEn_Set : FunctionCaller  FunctionPrototype=SecRwLtStLgrstInwdOtwdEn_Set(data)  InputArgumentSpecifications=uint8(1)
  wires:
  Constant/1 -> SecRwLtStLgrstInwdOtwdEn_Set/1

== system BigFour6sStEnCtrl/BigFour6sStEnCtrl_Cal_sys/Subsystem/If Action Subsystem15 ==
  note: Delete block
  Action Port : ActionPort  ActionType=else
  Constant : Constant  Value=24  OutDataTypeStr=uint8
  SecRwLtStLgrstUpwdDnwdEn_Clear : FunctionCaller  FunctionPrototype=SecRwLtStLgrstUpwdDnwdEn_Clear(data)  InputArgumentSpecifications=uint8(1)
  wires:
  Constant/1 -> SecRwLtStLgrstUpwdDnwdEn_Clear/1

== system BigFour6sStEnCtrl/BigFour6sStEnCtrl_Cal_sys/Subsystem/If Action Subsystem16 ==
  note: Delete block
  Action Port : ActionPort  ActionType=then
  Constant : Constant  Value=24  OutDataTypeStr=uint8
  SecRwLtStLgrstUpwdDnwdEn_Set : FunctionCaller  FunctionPrototype=SecRwLtStLgrstUpwdDnwdEn_Set(data)  InputArgumentSpecifications=uint8(1)
  wires:
  Constant/1 -> SecRwLtStLgrstUpwdDnwdEn_Set/1

== system BigFour6sStEnCtrl/BigFour6sStEnCtrl_Cal_sys/Subsystem/If Action Subsystem17 ==
  note: Delete block
  Action Port : ActionPort  ActionType=else
  Constant : Constant  Value=24  OutDataTypeStr=uint8
  ZeroLEn_Clear : FunctionCaller  FunctionPrototype=ZeroLEn_Clear(data)  InputArgumentSpecifications=uint8(1)
  wires:
  Constant/1 -> ZeroLEn_Clear/1

== system BigFour6sStEnCtrl/BigFour6sStEnCtrl_Cal_sys/Subsystem/If Action Subsystem18 ==
  note: Delete block
  Action Port : ActionPort  ActionType=then
  Constant : Constant  Value=24  OutDataTypeStr=uint8
  ZeroLEn_Set : FunctionCaller  FunctionPrototype=ZeroLEn_Set(data)  InputArgumentSpecifications=uint8(1)
  wires:
  Constant/1 -> ZeroLEn_Set/1

== system BigFour6sStEnCtrl/BigFour6sStEnCtrl_Cal_sys/Subsystem/If Action Subsystem19 ==
  note: Delete block
  Action Port : ActionPort  ActionType=else
  Constant : Constant  Value=24  OutDataTypeStr=uint8
  SecRwRtStLgrstInwdOtwdEn_Clear : FunctionCaller  FunctionPrototype=SecRwRtStLgrstInwdOtwdEn_Clear(data)  InputArgumentSpecifications=uint8(1)
  wires:
  Constant/1 -> SecRwRtStLgrstInwdOtwdEn_Clear/1

== system BigFour6sStEnCtrl/BigFour6sStEnCtrl_Cal_sys/Subsystem/If Action Subsystem20 ==
  note: Delete block
  Action Port : ActionPort  ActionType=then
  Constant : Constant  Value=24  OutDataTypeStr=uint8
  SecRwRtStLgrstInwdOtwdEn_Set : FunctionCaller  FunctionPrototype=SecRwRtStLgrstInwdOtwdEn_Set(data)  InputArgumentSpecifications=uint8(1)
  wires:
  Constant/1 -> SecRwRtStLgrstInwdOtwdEn_Set/1

== system BigFour6sStEnCtrl/BigFour6sStEnCtrl_Cal_sys/Subsystem/If Action Subsystem21 ==
  note: Delete block
  Action Port : ActionPort  ActionType=else
  Constant : Constant  Value=24  OutDataTypeStr=uint8
  SecRwRtStLgrstUpwdDnwdEn_Clear : FunctionCaller  FunctionPrototype=SecRwRtStLgrstUpwdDnwdEn_Clear(data)  InputArgumentSpecifications=uint8(1)
  wires:
  Constant/1 -> SecRwRtStLgrstUpwdDnwdEn_Clear/1

== system BigFour6sStEnCtrl/BigFour6sStEnCtrl_Cal_sys/Subsystem/If Action Subsystem22 ==
  note: Delete block
  Action Port : ActionPort  ActionType=then
  Constant : Constant  Value=24  OutDataTypeStr=uint8
  SecRwRtStLgrstUpwdDnwdEn_Set : FunctionCaller  FunctionPrototype=SecRwRtStLgrstUpwdDnwdEn_Set(data)  InputArgumentSpecifications=uint8(1)
  wires:
  Constant/1 -> SecRwRtStLgrstUpwdDnwdEn_Set/1

== system BigFour6sStEnCtrl/BigFour6sStEnCtrl_Cal_sys/Subsystem/If Action Subsystem23 ==
  note: Delete block
  Action Port : ActionPort  ActionType=else
  Constant : Constant  Value=24  OutDataTypeStr=uint8
  ZeroREn_Clear : FunctionCaller  FunctionPrototype=ZeroREn_Clear(data)  InputArgumentSpecifications=uint8(1)
  wires:
  Constant/1 -> ZeroREn_Clear/1

== system BigFour6sStEnCtrl/BigFour6sStEnCtrl_Cal_sys/Subsystem/If Action Subsystem24 ==
  note: Delete block
  Action Port : ActionPort  ActionType=then
  Constant : Constant  Value=24  OutDataTypeStr=uint8
  ZeroREn_Set : FunctionCaller  FunctionPrototype=ZeroREn_Set(data)  InputArgumentSpecifications=uint8(1)
  wires:
  Constant/1 -> ZeroREn_Set/1

== system BigFour6sStEnCtrl/BigFour6sStEnCtrl_Cal_sys/Subsystem/If Action Subsystem25 ==
  note: Delete block
  Action Port : ActionPort  ActionType=then
  Constant : Constant  Value=24  OutDataTypeStr=uint8
  SecRwLtStBkReclnEn_Set : FunctionCaller  FunctionPrototype=SecRwLtStBkReclnEn_Set(data)  InputArgumentSpecifications=uint8(1)
  wires:
  Constant/1 -> SecRwLtStBkReclnEn_Set/1

== system BigFour6sStEnCtrl/BigFour6sStEnCtrl_Cal_sys/Subsystem/If Action Subsystem26 ==
  note: Delete block
  Action Port : ActionPort  ActionType=then
  Constant : Constant  Value=24  OutDataTypeStr=uint8
  SecRwLtStBkReclnEn_Clear : FunctionCaller  FunctionPrototype=SecRwLtStBkReclnEn_Clear(data)  InputArgumentSpecifications=uint8(1)
  wires:
  Constant/1 -> SecRwLtStBkReclnEn_Clear/1

== system BigFour6sStEnCtrl/BigFour6sStEnCtrl_Cal_sys/Subsystem/If Action Subsystem27 ==
  note: Delete block
  Action Port : ActionPort  ActionType=then
  Constant : Constant  Value=24  OutDataTypeStr=uint8
  SecRwRtStBkReclnEn_Set : FunctionCaller  FunctionPrototype=SecRwRtStBkReclnEn_Set(data)  InputArgumentSpecifications=uint8(1)
  wires:
  Constant/1 -> SecRwRtStBkReclnEn_Set/1

== system BigFour6sStEnCtrl/BigFour6sStEnCtrl_Cal_sys/Subsystem/If Action Subsystem28 ==
  note: Delete block
  Action Port : ActionPort  ActionType=then
  Constant : Constant  Value=24  OutDataTypeStr=uint8
  SecRwRtStBkReclnEn_Clear : FunctionCaller  FunctionPrototype=SecRwRtStBkReclnEn_Clear(data)  InputArgumentSpecifications=uint8(1)
  wires:
  Constant/1 -> SecRwRtStBkReclnEn_Clear/1

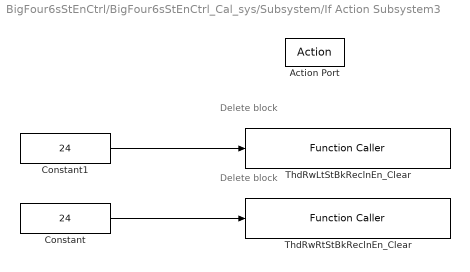
== system BigFour6sStEnCtrl/BigFour6sStEnCtrl_Cal_sys/Subsystem/If Action Subsystem3 ==
  note: Delete block
  note: Delete block
  Action Port : ActionPort  ActionType=else
  Constant : Constant  Value=24  OutDataTypeStr=uint8
  Constant1 : Constant  Value=24  OutDataTypeStr=uint8
  ThdRwLtStBkReclnEn_Clear : FunctionCaller  FunctionPrototype=ThdRwLtStBkReclnEn_Clear(data)  InputArgumentSpecifications=uint8(1)
  ThdRwRtStBkReclnEn_Clear : FunctionCaller  FunctionPrototype=ThdRwRtStBkReclnEn_Clear(data)  InputArgumentSpecifications=uint8(1)
  wires:
  Constant1/1 -> ThdRwLtStBkReclnEn_Clear/1
  Constant/1 -> ThdRwRtStBkReclnEn_Clear/1

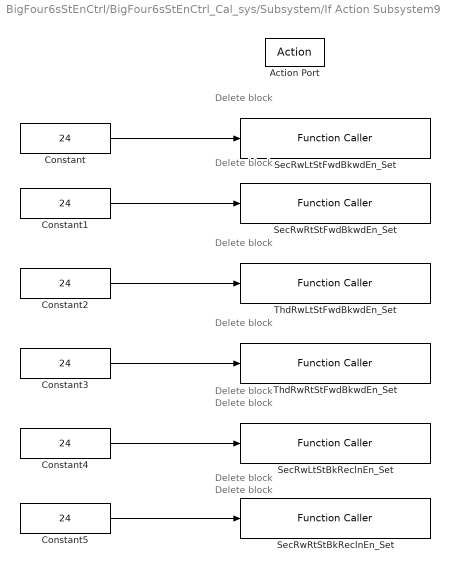
== system BigFour6sStEnCtrl/BigFour6sStEnCtrl_Cal_sys/Subsystem/If Action Subsystem9 ==
  note: Delete block
  note: Delete block
  note: Delete block
  note: Delete block
  note: Delete block
  note: Delete block
  note: Delete block
  note: Delete block
  Action Port : ActionPort  ActionType=then
  Constant{,1..5} (6 alike) : Constant  Value=24  OutDataTypeStr=uint8
  SecRwLtStBkReclnEn_Set : FunctionCaller  FunctionPrototype=SecRwLtStBkReclnEn_Set(data)  InputArgumentSpecifications=uint8(1)
  SecRwLtStFwdBkwdEn_Set : FunctionCaller  FunctionPrototype=SecRwLtStFwdBkwdEn_Set(data)  InputArgumentSpecifications=uint8(1)
  SecRwRtStBkReclnEn_Set : FunctionCaller  FunctionPrototype=SecRwRtStBkReclnEn_Set(data)  InputArgumentSpecifications=uint8(1)
  SecRwRtStFwdBkwdEn_Set : FunctionCaller  FunctionPrototype=SecRwRtStFwdBkwdEn_Set(data)  InputArgumentSpecifications=uint8(1)
  ThdRwLtStFwdBkwdEn_Set : FunctionCaller  FunctionPrototype=ThdRwLtStFwdBkwdEn_Set(data)  InputArgumentSpecifications=uint8(1)
  ThdRwRtStFwdBkwdEn_Set : FunctionCaller  FunctionPrototype=ThdRwRtStFwdBkwdEn_Set(data)  InputArgumentSpecifications=uint8(1)
  wires:
  Constant/1 -> SecRwLtStFwdBkwdEn_Set/1
  Constant1/1 -> SecRwRtStFwdBkwdEn_Set/1
  Constant2/1 -> ThdRwLtStFwdBkwdEn_Set/1
  Constant3/1 -> ThdRwRtStFwdBkwdEn_Set/1
  Constant4/1 -> SecRwLtStBkReclnEn_Set/1
  Constant5/1 -> SecRwRtStBkReclnEn_Set/1

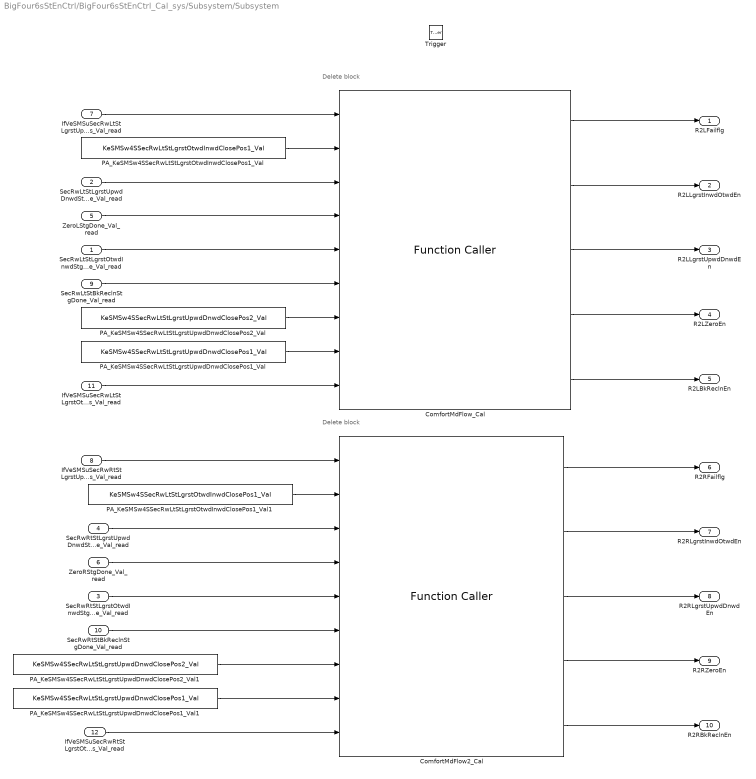
== system BigFour6sStEnCtrl/BigFour6sStEnCtrl_Cal_sys/Subsystem/Subsystem ==
  note: Delete block
  note: Delete block
  SecRwLtStLgrstOtwdInwdStgDone_Val_read : Inport
  SecRwLtStLgrstUpwdDnwdStgDone_Val_read : Inport  Port=2
  SecRwRtStLgrstOtwdInwdStgDone_Val_read : Inport  Port=3
  SecRwRtStLgrstUpwdDnwdStgDone_Val_read : Inport  Port=4
  ZeroLStgDone_Val_read : Inport  Port=5
  ZeroRStgDone_Val_read : Inport  Port=6
  IfVeSMSuSecRwLtStLgrstUpwdDnwdPos_Val_read : Inport  Port=7
  IfVeSMSuSecRwRtStLgrstUpwdDnwdPos_Val_read : Inport  Port=8
  SecRwLtStBkReclnStgDone_Val_read : Inport  Port=9
  SecRwRtStBkReclnStgDone_Val_read : Inport  Port=10
  IfVeSMSuSecRwLtStLgrstOtwdInwdPos_Val_read : Inport  Port=11
  IfVeSMSuSecRwRtStLgrstOtwdInwdPos_Val_read : Inport  Port=12
  Trigger : TriggerPort  TriggerType=function-call  VariantControl=Variant  PortDimensions=1
  ComfortMdFlow2_Cal : FunctionCaller  FunctionPrototype=[Failflg,LgrstInwdOtwdEn,LgrstUpwdDnwdEn,ZeroEn,BkReclnEn] = ComfortMdFlow2_Cal(LgrstUpwdDnwdPos,LgrstUpwdDnwdClosePos1,LgrstUpwdStgDone,ZeroStgDone,LgrstInwdStgDone,BkReclnStgDone,LgrstUpwdDnwdClosePos2,LgrstInwdOtwdClosePos1,LgrstInwdOtwdPos)  InputArgumentSpecifications=uint16(1), uint16(1), boolean(true), boolean(true), boolean(true), boolean(true), uint16(1), uint16(1), uint16(1)  OutputArgumentSpecifications=boolean(true), boolean(true), boolean(true), boolean(true), boolean(true)
  ComfortMdFlow_Cal : FunctionCaller  FunctionPrototype=[Failflg,LgrstInwdOtwdEn,LgrstUpwdDnwdEn,ZeroEn,BkReclnEn] = ComfortMdFlow_Cal(LgrstUpwdDnwdPos,LgrstUpwdDnwdClosePos1,LgrstUpwdStgDone,ZeroStgDone,LgrstInwdStgDone,BkReclnStgDone,LgrstUpwdDnwdClosePos2,LgrstInwdOtwdClosePos1,LgrstInwdOtwdPos)  InputArgumentSpecifications=uint16(1), uint16(1), boolean(true), boolean(true), boolean(true), boolean(true), uint16(1), uint16(1), uint16(1)  OutputArgumentSpecifications=boolean(true), boolean(true), boolean(true), boolean(true), boolean(true)
  PA_KeSMSw4SSecRwLtStLgrstOtwdInwdClosePos1_Val : Constant  Value=KeSMSw4SSecRwLtStLgrstOtwdInwdClosePos1_Val
  PA_KeSMSw4SSecRwLtStLgrstOtwdInwdClosePos1_Val1 : Constant  Value=KeSMSw4SSecRwLtStLgrstOtwdInwdClosePos1_Val
  PA_KeSMSw4SSecRwLtStLgrstUpwdDnwdClosePos1_Val : Constant  Value=KeSMSw4SSecRwLtStLgrstUpwdDnwdClosePos1_Val
  PA_KeSMSw4SSecRwLtStLgrstUpwdDnwdClosePos1_Val1 : Constant  Value=KeSMSw4SSecRwLtStLgrstUpwdDnwdClosePos1_Val
  PA_KeSMSw4SSecRwLtStLgrstUpwdDnwdClosePos2_Val : Constant  Value=KeSMSw4SSecRwLtStLgrstUpwdDnwdClosePos2_Val
  PA_KeSMSw4SSecRwLtStLgrstUpwdDnwdClosePos2_Val1 : Constant  Value=KeSMSw4SSecRwLtStLgrstUpwdDnwdClosePos2_Val
  R2LFailflg : Outport
  R2LLgrstInwdOtwdEn : Outport  Port=2
  R2LLgrstUpwdDnwdEn : Outport  Port=3
  R2LZeroEn : Outport  Port=4
  R2LBkReclnEn : Outport  Port=5
  R2RFailflg : Outport  Port=6
  R2RLgrstInwdOtwdEn : Outport  Port=7
  R2RLgrstUpwdDnwdEn : Outport  Port=8
  R2RZeroEn : Outport  Port=9
  R2RBkReclnEn : Outport  Port=10
  wires:
  SecRwRtStLgrstUpwdDnwdStgDone_Val_read/1 -> ComfortMdFlow2_Cal/3
  SecRwRtStLgrstOtwdInwdStgDone_Val_read/1 -> ComfortMdFlow2_Cal/5
  IfVeSMSuSecRwRtStLgrstUpwdDnwdPos_Val_read/1 -> ComfortMdFlow2_Cal/1
  ComfortMdFlow_Cal/1 -> R2LFailflg/1
  PA_KeSMSw4SSecRwLtStLgrstOtwdInwdClosePos1_Val/1 -> ComfortMdFlow_Cal/2
  ZeroRStgDone_Val_read/1 -> ComfortMdFlow2_Cal/4
  SecRwLtStLgrstOtwdInwdStgDone_Val_read/1 -> ComfortMdFlow_Cal/5
  SecRwLtStLgrstUpwdDnwdStgDone_Val_read/1 -> ComfortMdFlow_Cal/3
  ZeroLStgDone_Val_read/1 -> ComfortMdFlow_Cal/4
  IfVeSMSuSecRwLtStLgrstUpwdDnwdPos_Val_read/1 -> ComfortMdFlow_Cal/1
  SecRwLtStBkReclnStgDone_Val_read/1 -> ComfortMdFlow_Cal/6
  SecRwRtStBkReclnStgDone_Val_read/1 -> ComfortMdFlow2_Cal/6
  ComfortMdFlow_Cal/2 -> R2LLgrstInwdOtwdEn/1
  ComfortMdFlow_Cal/3 -> R2LLgrstUpwdDnwdEn/1
  ComfortMdFlow_Cal/4 -> R2LZeroEn/1
  ComfortMdFlow_Cal/5 -> R2LBkReclnEn/1
  ComfortMdFlow2_Cal/5 -> R2RBkReclnEn/1
  ComfortMdFlow2_Cal/4 -> R2RZeroEn/1
  ComfortMdFlow2_Cal/3 -> R2RLgrstUpwdDnwdEn/1
  ComfortMdFlow2_Cal/2 -> R2RLgrstInwdOtwdEn/1
  ComfortMdFlow2_Cal/1 -> R2RFailflg/1
  PA_KeSMSw4SSecRwLtStLgrstUpwdDnwdClosePos2_Val1/1 -> ComfortMdFlow2_Cal/7
  PA_KeSMSw4SSecRwLtStLgrstUpwdDnwdClosePos1_Val1/1 -> ComfortMdFlow2_Cal/8
  IfVeSMSuSecRwRtStLgrstOtwdInwdPos_Val_read/1 -> ComfortMdFlow2_Cal/9
  PA_KeSMSw4SSecRwLtStLgrstUpwdDnwdClosePos2_Val/1 -> ComfortMdFlow_Cal/7
  PA_KeSMSw4SSecRwLtStLgrstUpwdDnwdClosePos1_Val/1 -> ComfortMdFlow_Cal/8
  IfVeSMSuSecRwLtStLgrstOtwdInwdPos_Val_read/1 -> ComfortMdFlow_Cal/9
  PA_KeSMSw4SSecRwLtStLgrstOtwdInwdClosePos1_Val1/1 -> ComfortMdFlow2_Cal/2

== stateflow chart BigFour6sStEnCtrl/BigFour6sStEnCtrl_Cal_sys/Subsystem/Chart ==
  (default) -> (junction 95) : {
      | Stage1En = 0;
      | Stage2En = 0;
      | }
  (junction 95) -> (junction 97) [order 1] : [!Stage1Done]
  (junction 95) -> (junction 101) [order 2]
  (junction 97) -> (junction 208) : {
      | TrigComfortMd;
      | Stage1En =1 ;
      | }
  (junction 101) -> (junction 104) [order 1] : [!Stage2Done]
  (junction 101) -> (junction 109) [order 2]
  (junction 104) -> (junction 106) : {Stage2En = 1;}
  (junction 106) -> (junction 109)
  (junction 208) -> (junction 106)
  (junction 109) -> (junction 196)
  data: Stage1Done input boolean; Stage2Done input boolean; Stage2En output boolean; Stage1En output boolean
  events: TrigComfortMd output FUNCTION_CALL_EVENT
